simulink model "Model_Predictive_Control_R2015a"  (R2015a)
settings: Solver=ode45  StartTime=0.0  StopTime=500  RelTol=1e-3
StartFcn:
  | clear all
libraries: simulink x1, realtime_pacer_lib x1
settings Model: Creator=johnh  LastModifiedBy=John Hedengren
settings DataIOCC: LimitDataPoints=off  SaveFormat=Dataset
settings HardwareCC: ProdBitPerPointer=64  ProdLargestAtomicFloat=Float  ProdIntDivRoundTo=Zero  ProdEndianess=LittleEndian  ProdHWDeviceType=Specified
settings ModelReferenceCC: PropagateSignalLabelsOutOfModel=on

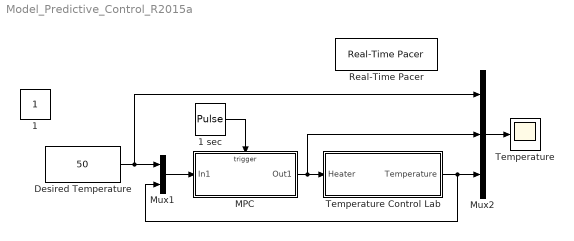
== system Model_Predictive_Control_R2015a ==
  1 sec : DiscretePulseGenerator  PulseType=Time based  Period=1  PulseWidth=5
  Desired Temperature : simulink/Math Operations/Slider Gain  gain=50  low=0  high=100
  MPC : Subsystem  TreatAsAtomicUnit=on
  Mux1 : Mux  Inputs=2
  Mux2 : Mux  Inputs=3
  Real-Time Pacer : realtime_pacer_lib/Real-Time Pacer  simTimePerRealTime=1
  Temperature : Scope
      settings: TimeRange=auto  MaxDataPoints=5000  SaveToWorkspace=off  YMin=-12.5  YMax=112.5  SampleTime=-1
  Temperature Control Lab : Subsystem
  1 : Constant  IOType=siggen
  wires:
  Temperature Control Lab/1(Temperature) -> Mux2/3, Mux1/2
  1 sec/1 -> MPC/Trigger
  MPC/1(Out1) -> Mux2/2, Temperature Control Lab/1(Heater)
  Mux1/1 -> MPC/1(In1)
  Desired Temperature/1 -> Mux2/1, Mux1/1
  Mux2/1 -> Temperature/1

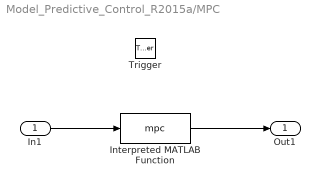
== system Model_Predictive_Control_R2015a/MPC ==
  In1 : Inport  LatchByDelayingOutsideSignal=on
  Trigger : TriggerPort
  Interpreted MATLAB Function : MATLABFcn  MATLABFcn=mpc  OutputDimensions=1
  Out1 : Outport  InitialOutput=0
  wires:
  In1/1 -> Interpreted MATLAB Function/1
  Interpreted MATLAB Function/1 -> Out1/1

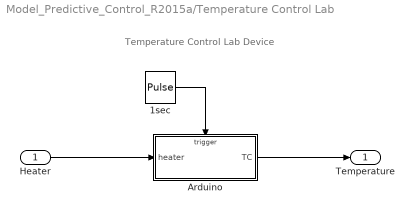
== system Model_Predictive_Control_R2015a/Temperature Control Lab ==
  note: Temperature Control Lab Device
  Heater : Inport
  1sec : DiscretePulseGenerator  PulseType=Time based  Period=1  PulseWidth=50
  Arduino : Subsystem  TreatAsAtomicUnit=on
  Temperature : Outport
  wires:
  1sec/1 -> Arduino/Trigger
  Arduino/1(TC) -> Temperature/1
  Heater/1 -> Arduino/1(heater)

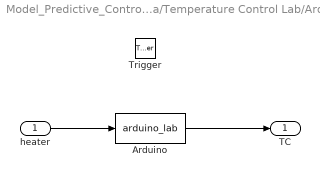
== system Model_Predictive_Control_R2015a/Temperature Control Lab/Arduino ==
  heater : Inport  LatchByDelayingOutsideSignal=on
  Trigger : TriggerPort
  Arduino : MATLABFcn  MATLABFcn=arduino_lab
  TC : Outport  InitialOutput=23
  wires:
  heater/1 -> Arduino/1
  Arduino/1 -> TC/1
